simulink subsystem "guidance_command_calculator"  (R2025b)
settings: Solver=VariableStepAuto  StartTime=0.0  StopTime=10.0  RelTol=1e-3
settings Model: Creator=aksaf  LastModifiedBy=aksaf

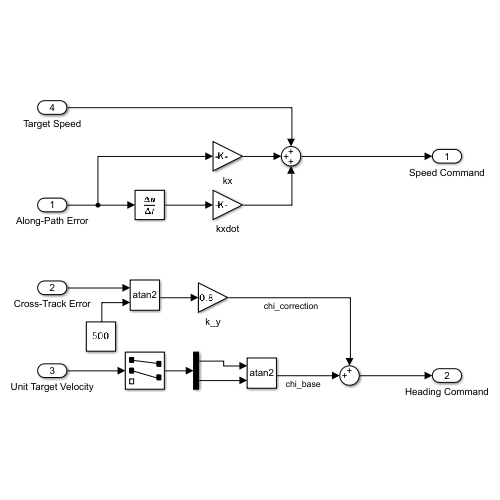
[thumbnail: Simulink's stored preview of the top-level diagram]
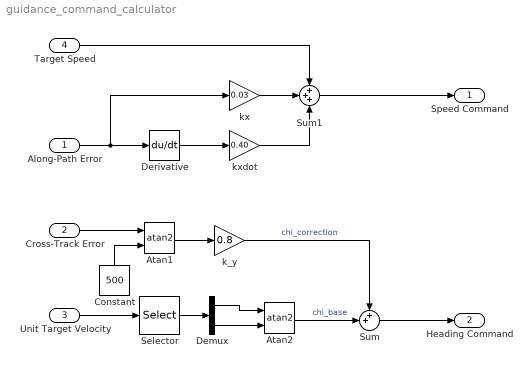
== system guidance_command_calculator ==
  Along-Path Error : Inport
  Cross-Track Error : Inport  Port=2
  Unit Target Velocity : Inport  Port=3
  Target Speed : Inport  Port=4
  Atan1 : Trigonometry  Operator=atan2
  Atan2 : Trigonometry  Operator=atan2
  Constant : Constant  Value=500
  Demux : Demux  Outputs=2
  Derivative : Derivative
  Selector : Selector  InputPortWidth=3  IndexOptions=Index vector (dialog)  Indices=[1 2]  OutputSizes=1
  Sum : Sum  Inputs=++|
  Sum1 : Sum  Inputs=+++
  k_y : Gain  Gain=0.8
  kx : Gain  Gain=0.03
  kxdot : Gain  Gain=0.40
  Speed Command : Outport
  Heading Command : Outport  Port=2
  wires:
  Unit Target Velocity/1 -> Selector/1
  Selector/1 -> Demux/1
  Demux/1 -> Atan2/1
  Demux/2 -> Atan2/2
  Constant/1 -> Atan1/2
  Cross-Track Error/1 -> Atan1/1
  Atan1/1 -> k_y/1
  k_y/1 -> Sum/1  "chi_correction"
  Atan2/1 -> Sum/2  "chi_base"
  Sum/1 -> Heading Command/1
  Along-Path Error/1 -> kx/1, Derivative/1
  Derivative/1 -> kxdot/1
  kx/1 -> Sum1/2
  kxdot/1 -> Sum1/3
  Target Speed/1 -> Sum1/1
  Sum1/1 -> Speed Command/1
